simulink model "Probe1"  (R2017b)
settings: Solver=FixedStepDiscrete  StartTime=0.0  StopTime=19.8  FixedStep=0.200000  RelTol=1e-3  EnableMultiTasking=on
settings Model: Creator=hbourbou  LastModifiedBy=hbourbou
settings DataIOCC: ExternalInput=input_dataset  LimitDataPoints=on  SaveState=on
settings OptimizationCC: LifeSpan=inf
settings DebuggingCC: AlgebraicLoopMsg=error  SFUnexpectedBacktrackingDiag=warning  SFNoUnconditionalDefaultTransitionDiag=warning  SFExecutionAtInitializationDiag=none
settings HardwareCC: ProdBitPerPointer=32  ProdBitPerSizeT=32  ProdBitPerPtrDiffT=32  ProdLargestAtomicFloat=None  ProdIntDivRoundTo=Undefined  ProdEndianess=Unspecified  ProdWordSize=32  ProdHWDeviceType=32-bit Generic
settings ModelReferenceCC: PropagateSignalLabelsOutOfModel=off
settings CodeAppCC: StateflowObjectComments=on
settings GRTTargetCC: TargetLangStandard=C89/C90 (ANSI)  GeneratePreprocessorConditionals=Disable all  ExtMode=on
settings ConfigComp: CovMetricSettings=dw  CovHtmlReporting=on  CovSaveCumulativeToWorkspaceVar=on  CovSaveSingleToWorkspaceVar=on  CovExternalEMLEnable=off

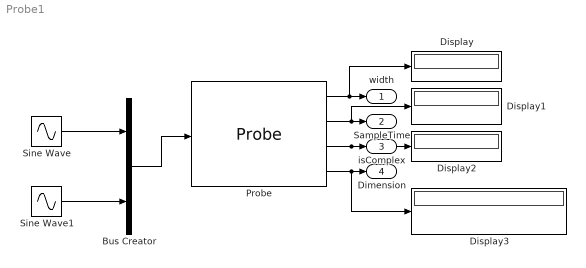
== system Probe1 ==
  Bus Creator : BusCreator  Inputs=2
  Display{,1..3} (4 alike) : Display
  Probe : Probe  ProbeSignalDimensions=on  ProbeWidthDataType=uint8  ProbeComplexityDataType=boolean  ProbeDimensionsDataType=uint8
  Sine Wave : Sin  SampleTime=0
  Sine Wave1 : Sin  SampleTime=0
  width : Outport
  SampleTime : Outport  Port=2
  isComplex : Outport  Port=3
  Dimension : Outport  Port=4
  wires:
  Probe/1 -> Display/1, width/1
  Probe/2 -> Display1/1, SampleTime/1
  Probe/3 -> Display2/1, isComplex/1
  Probe/4 -> Display3/1, Dimension/1
  Sine Wave/1 -> Bus Creator/1
  Sine Wave1/1 -> Bus Creator/2
  Bus Creator/1 -> Probe/1
